simulink model "Sim"  (R2018a)
settings: Solver=FixedStepAuto  StartTime=0.0  StopTime=EndTime  FixedStep=dt  RelTol=1e-3
values from neighbouring files (symbols this model uses):
  A = pi/4*D^2    (= 1086.86539444)    [ParametricResonance_Regular.m]    (also in ParametricResonance_Spectrum.m)
  C = [C3,C5]'    [ParametricResonance_Regular.m]    (also in ParametricResonance_Spectrum.m)
  DeltaV = A*Df    (= 215308.034638)    [ParametricResonance_Regular.m]    (also in ParametricResonance_Spectrum.m)
  g = 9.81    [ParametricResonance_Regular.m]    (also in ParametricResonance_Spectrum.m)
  GM = 10.1    [ParametricResonance_Regular.m]    (also in ParametricResonance_Spectrum.m)
  Heave1 = 0    [ParametricResonance_Regular.m]    (also in ParametricResonance_Spectrum.m)
  Hg = Df-KG    (= 109.1)    [ParametricResonance_Regular.m]    (also in ParametricResonance_Spectrum.m)
  I = [m+A33,I55+A55]'    [ParametricResonance_Regular.m]    (also in ParametricResonance_Spectrum.m)
  Pitch1 = 0    [ParametricResonance_Regular.m]    (also in ParametricResonance_Spectrum.m)
  rho = 1000    [ParametricResonance_Regular.m]    (also in ParametricResonance_Spectrum.m = 1003)
libraries: simulink x1
settings Model: Creator=root  LastModifiedBy=josh

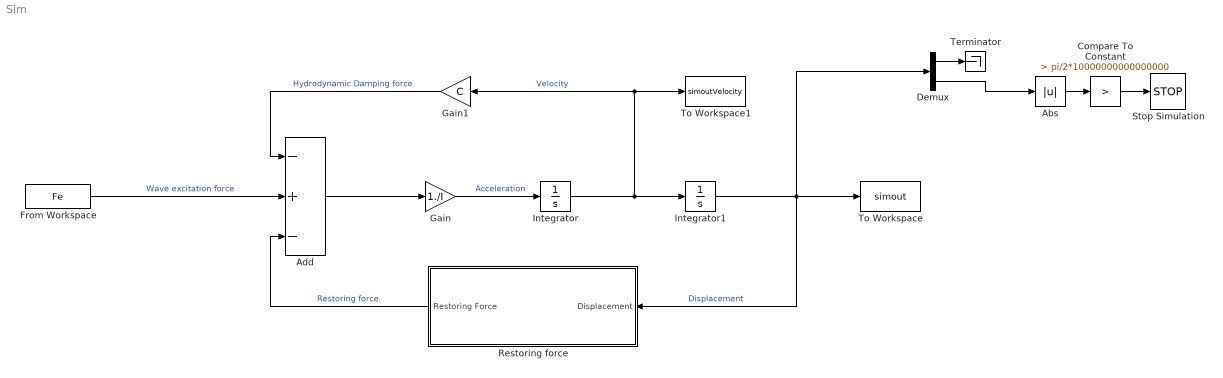
== system Sim ==
  Abs : Abs
  Add : Sum  Inputs=-+-
  Compare To Constant : simulink/Logic and Bit Operations/Compare To Constant  relop=>  const=pi/2*10000000000000000  OutDataTypeStr=boolean
  Demux : Demux  Outputs=2
  From Workspace : FromWorkspace  VariableName=Fe  SampleTime=0
  Gain : Gain  Gain=1./I
  Gain1 : Gain  Gain=C
  Integrator : Integrator
  Integrator1 : Integrator  InitialCondition=[Heave1,Pitch1]
  Restoring force : Subsystem
  Stop Simulation : Stop
  Terminator : Terminator
  To Workspace : ToWorkspace  VariableName=simout  SaveFormat=Timeseries  SampleTime=-1
  To Workspace1 : ToWorkspace  VariableName=simoutVelocity  SaveFormat=Timeseries  SampleTime=-1
  wires:
  Add/1 -> Gain/1
  Gain/1 -> Integrator/1  "Acceleration"
  Integrator/1 -> To Workspace1/1, Gain1/1, Integrator1/1  "Velocity"
  Gain1/1 -> Add/1  "Hydrodynamic Damping force"
  Restoring force/1(Restoring Force) -> Add/3  "Restoring force"
  Compare To Constant/1 -> Stop Simulation/1
  Abs/1 -> Compare To Constant/1
  Integrator1/1 -> Demux/1, To Workspace/1, Restoring force/1(Displacement)  "Displacement"
  Demux/2 -> Abs/1
  Demux/1 -> Terminator/1
  From Workspace/1 -> Add/2  "Wave excitation force"

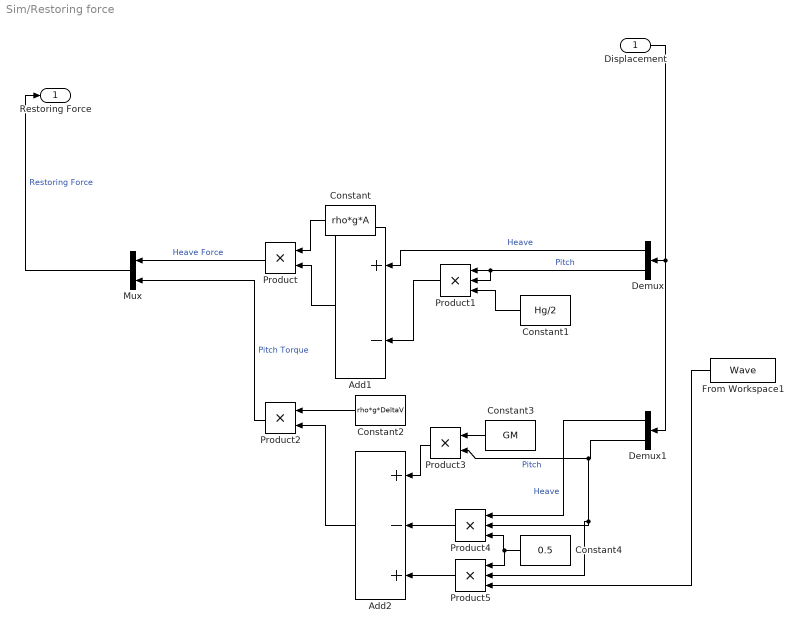
== system Sim/Restoring force ==
  Displacement : Inport
  Add1 : Sum  Inputs=+-
  Add2 : Sum  Inputs=+-+
  Constant : Constant  Value=rho*g*A
  Constant1 : Constant  Value=Hg/2
  Constant2 : Constant  Value=rho*g*DeltaV
  Constant3 : Constant  Value=GM
  Constant4 : Constant  Value=0.5
  Demux : Demux  Outputs=2
  Demux1 : Demux  Outputs=2
  From Workspace1 : FromWorkspace  VariableName=Wave  SampleTime=0
  Mux : Mux  Inputs=2
  Product : Product
  Product1 : Product  Inputs=3
  Product2 : Product
  Product3 : Product
  Product4 : Product  Inputs=3
  Product5 : Product  Inputs=3
  Restoring Force : Outport
  wires:
  Add2/1 -> Product2/2
  Constant3/1 -> Product3/1
  Constant1/1 -> Product1/3
  Product/1 -> Mux/1  "Heave Force"
  Demux/2 -> Product1/2, Product1/1  "Pitch"
  Demux1/2 -> Product5/2, Product4/2, Product3/2  "Pitch"
  Constant/1 -> Product/1
  Product4/1 -> Add2/2
  Product1/1 -> Add1/2
  Mux/1 -> Restoring Force/1  "Restoring Force"
  Product5/1 -> Add2/3
  Constant4/1 -> Product5/1, Product4/3
  From Workspace1/1 -> Product5/3
  Demux1/1 -> Product4/1  "Heave"
  Product3/1 -> Add2/1
  Add1/1 -> Product/2
  Product2/1 -> Mux/2  "Pitch Torque"
  Constant2/1 -> Product2/1
  Demux/1 -> Add1/1  "Heave"
  Displacement/1 -> Demux1/1, Demux/1
